simulink subsystem "Day2_Scenario_2_3"  (R2024a)
settings: Solver=VariableStepAuto  StartTime=0.0  StopTime=10.0  RelTol=1e-3
libraries: CarMaker4SL x5
settings Model: Creator=junhyung.cha  LastModifiedBy=User

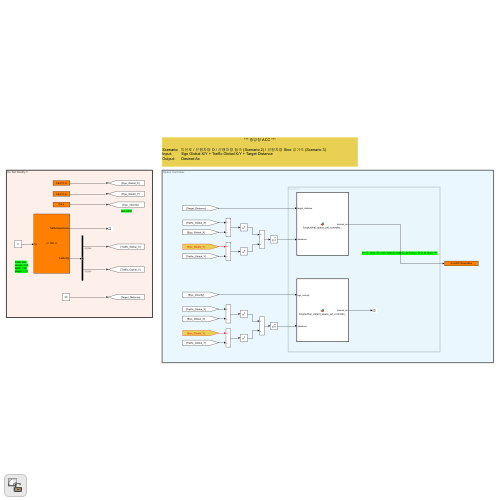
[thumbnail: Simulink's stored preview of the top-level diagram]
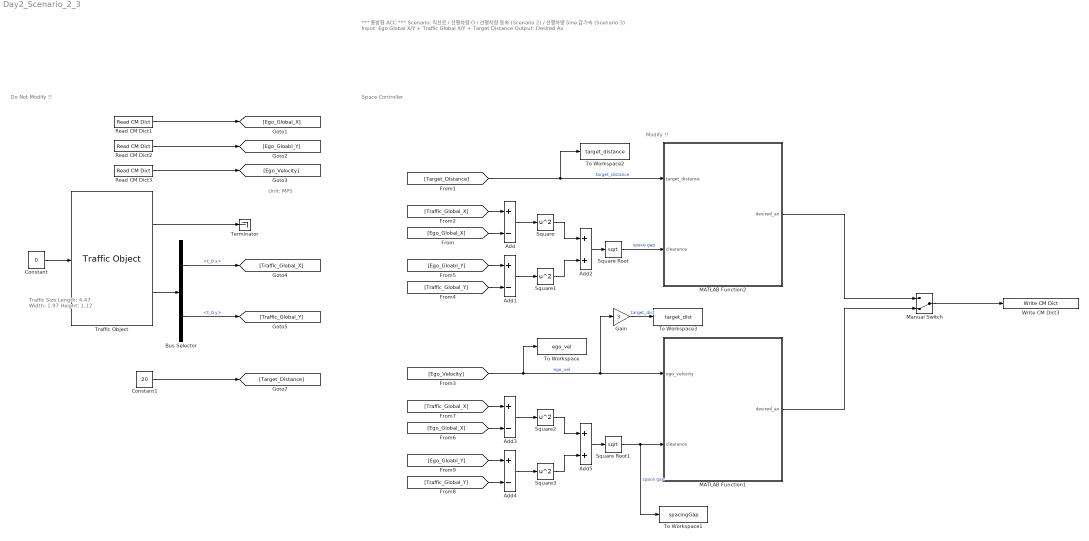
== system Day2_Scenario_2_3 ==
  note: Space Controller
  note: Modify !!
  note: Do Not Modify !!
  note: Traffic Size
      | Length: 4.47
      | Width: 1.97
      | Height: 1.12
  note: *** 종방향 ACC ***
      |
      | Scenario: 직선로 / 선행차량 O / 선행차량 등속 (Scenario 2) / 선행차량 Sine 감가속 (Scenario 3)
      | Input: Ego Global X/Y + Traffic Global X/Y + Target Distance
      | Output: Desired Ax
  note: Unit: MPS
  Add{,1,3..4} (4 alike) : Sum  Inputs=+-
  Add2 : Sum
  Add5 : Sum
  Bus Selector : BusSelector  OutputSignals=t_0 x,t_0 y
  Constant : Constant  Value=0
  Constant1 : Constant  Value=20
  Gain : Gain  Gain=3
  MATLAB Function1 : MATLAB Function  TreatAsAtomicUnit=on
  MATLAB Function2 : MATLAB Function  TreatAsAtomicUnit=on
  Manual Switch : ManualSwitch  CurrentSetting=0
  Read CM Dict1 : CarMaker4SL/Read CM Dict  xname=Car.Fr1.tx  xsync=off  xstime=Inherited
  Read CM Dict2 : CarMaker4SL/Read CM Dict  xname=Car.Fr1.ty  xsync=off  xstime=Inherited
  Read CM Dict3 : CarMaker4SL/Read CM Dict  xname=Car.v  xsync=off  xstime=Inherited
  Square{,1..3} (4 alike) : Math  Operator=square
  Square Root : Sqrt
  Square Root1 : Sqrt
  Terminator : Terminator
  To Workspace : ToWorkspace  VariableName=ego_vel  SaveFormat=Timeseries  SampleTime=-1
  To Workspace1 : ToWorkspace  VariableName=spacingGap  SaveFormat=Timeseries  SampleTime=-1
  To Workspace2 : ToWorkspace  VariableName=target_distance  SaveFormat=Timeseries  SampleTime=-1
  To Workspace3 : ToWorkspace  VariableName=target_dist  SaveFormat=Timeseries  SampleTime=-1
  Traffic Object : CarMaker4SL/Traffic Object  xname=T00  ximode=Traffic Id  xstime=Inherited
      settings: SourceProductName=CarMaker4SL
  Write CM Dict3 : CarMaker4SL/Write CM Dict  xname=AccelCtrl.DesiredAx  xsync=off
  wires:
  Read CM Dict2/1 -> [Ego_Gloabl_Y]
  Read CM Dict1/1 -> [Ego_Global_X]
  Constant/1 -> Traffic Object/1
  Traffic Object/2 -> Bus Selector/1
  Traffic Object/1 -> Terminator/1
  Bus Selector/1 -> [Traffic_Global_X]  "<t_0 x>"
  Bus Selector/2 -> [Traffic_Global_Y]  "<t_0 y>"
  Square Root/1 -> MATLAB Function2/2(clearance)  "space gap"
  Constant1/1 -> [Target_Distance]
  [Ego_Global_X] -> Add/2
  [Traffic_Global_X] -> Add/1
  [Traffic_Global_Y] -> Add1/2
  [Ego_Gloabl_Y] -> Add1/1
  Add1/1 -> Square1/1
  Add2/1 -> Square Root/1
  Square/1 -> Add2/1
  Square1/1 -> Add2/2
  [Target_Distance] -> MATLAB Function2/1(target_distance), To Workspace2/1  "target_distance"
  Add/1 -> Square/1
  Read CM Dict3/1 -> [Ego_Velocity]
  [Ego_Velocity] -> MATLAB Function1/1(ego_velocity), Gain/1, To Workspace/1  "ego_vel"
  Add3/1 -> Square2/1
  Square3/1 -> Add5/2
  Square2/1 -> Add5/1
  Add5/1 -> Square Root1/1
  Add4/1 -> Square3/1
  [Ego_Gloabl_Y] -> Add4/1
  [Traffic_Global_Y] -> Add4/2
  [Traffic_Global_X] -> Add3/1
  [Ego_Global_X] -> Add3/2
  Square Root1/1 -> MATLAB Function1/2(clearance), To Workspace1/1  "space gap"
  Gain/1 -> To Workspace3/1  "target_dist"
  Manual Switch/1 -> Write CM Dict3/1
  MATLAB Function2/1(desired_ax) -> Manual Switch/1
  MATLAB Function1/1(desired_ax) -> Manual Switch/2

== matlab function Day2_Scenario_2_3/MATLAB Function1 ==
  settings: updateMethod=DISCRETE  sampleTime=0.05
  data: ego_velocity input; desired_ax output; clearance input
function desired_ax = longitudinal_variant_space_pd_controller_(ego_velocity, clearance)
    desired_ax = longitudinal_variant_space_pd_controller_mfile(ego_velocity, clearance);
end


function desired_ax = longitudinal_variant_space_pd_controller_mfile(ego_velocity, clearance)
    
    persistent error_prev
    dt = 0.05;
    time_gap = 3.0;
    target_distance = ego_velocity*time_gap;

    error = clearance - target_distance;
    
    if isempty(error_prev)
        error_prev = error;
    end

    Kp = 3.0;
    Kd = 1.0;

    P_term = Kp*error;
    D_term = Kd*(error - error_prev) / dt;
    
    desired_ax = (P_term + D_term);
    error_prev = error;
end

== matlab function Day2_Scenario_2_3/MATLAB Function2 ==
  settings: updateMethod=DISCRETE  sampleTime=0.05
  data: target_distance input; desired_ax output; clearance input
function desired_ax = longitudinal_space_pid_controller_(target_distance, clearance)
    desired_ax = longitudinal_space_pid_controller_mifle(target_distance, clearance);
end

function desired_ax = longitudinal_space_pid_controller_mifle(target_distance, clearance)
    persistent error_prev error_sum
    dt = 0.05;
    
    error = clearance - target_distance;
    
    if isempty(error_prev)
        error_prev = error;
    end

    if isempty(error_sum)
        error_sum = 0;
    else
        if error < 10
            error_sum = error_sum + error * dt;
        end
    end

    Kp = 1.5;
    Ki = 0.01;
    Kd = 2.0;

    P_term = Kp*error;
    I_term = Ki*error_sum;
    D_term = Kd*(error - error_prev) / dt;
    
    desired_ax = (P_term + I_term + D_term);
    error_prev = error;
end
